simulink model "Hybrid_BCI"  (Simulink 8.6)
settings: Solver=FixedStepDiscrete  StartTime=0.0  StopTime=260  FixedStep=1/256  RelTol=1e-3
undefined symbols (not defined in the file or in its folder): currentCFG_Hybrid_BCI_UB, UB
libraries: dspstat3 x6, gRTanalyze x5, dspbuff3 x5, simulink x2, Tools x1, instrumentlib x1, gUSBamplib x1
Description:
  | g.USBamp based SSVEP based BCI
  | 
  | Copyright g.tec medical engineering GmbH
settings Model: Creator=g.tec medical engineering GmbH  ModifiedByFormat=g.tec  LastModifiedBy=g.tec
settings DebuggingCC: FcnCallInpInsideContextMsg=UseLocalSettings

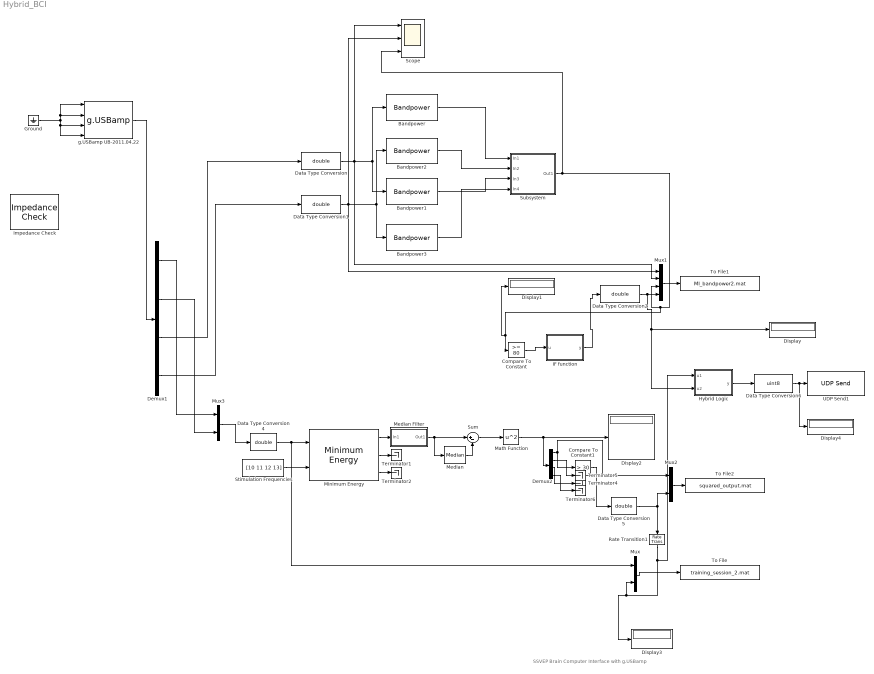
== system Hybrid_BCI ==
  note: SSVEP Brain Computer Interface with g.USBamp
  Bandpower : gRTanalyze/Bandpower  Order=5  LowerFreq=8  UpperFreq=12  WindowLength=128
  Bandpower1 : gRTanalyze/Bandpower  Order=5  LowerFreq=12  UpperFreq=30  WindowLength=128
  Bandpower2 : gRTanalyze/Bandpower  Order=5  LowerFreq=8  UpperFreq=12  WindowLength=128
  Bandpower3 : gRTanalyze/Bandpower  Order=5  LowerFreq=12  UpperFreq=30  WindowLength=128
  Compare To Constant : simulink/Logic and Bit Operations/Compare To Constant  relop=>=  const=80  OutDataTypeStr=boolean
  Compare To Constant1 : simulink/Logic and Bit Operations/Compare To Constant  relop=>  const=30  OutDataTypeStr=boolean
  Data Type Conversion{,1..2,4..5} (5 alike) : DataTypeConversion  OutDataTypeStr=double
  Data Type Conversion6 : DataTypeConversion  OutDataTypeStr=uint8
  Demux1 : Demux
  Demux2 : Demux
  Display{,1..4} (5 alike) : Display
  Ground : Ground
  Hybrid Logic : MATLAB Function  TreatAsAtomicUnit=on
  IF function : MATLAB Function  TreatAsAtomicUnit=on
  Impedance Check : Tools/Impedance Check
  Math Function : Math  Operator=square  SaturateOnIntegerOverflow=on
  Median : dspstat3/Median  sortAlg=Quick sort  directionMode=Entire input  dimension=1  outputDataTypeStr=Inherit: Same as accumulator  outputLastDataTypeStr=Inherit: Same as accumulator  outputMin=[]  outputMax=[]  accumDataTypeStr=Inherit: Same as product output  accumLastDataTypeStr=Inherit: Same as product output  roundingMode=Floor  overflowMode=off
      settings: allowOverrides=off
  Median Filter : Subsystem  mask(Moving Median Filter){buflen=10}
      mask prompts: buflen "Filter Length"
      mask help:
      | Smoothes the input channels over time by computing the median value for
      | the specified number of samples.
      mask init:
      | blockhandle = get_param(gcb,'Handle');
      | sysname = get(blockhandle,'Path');
      | syspath = [ sysname '/' ];
      | name = [ syspath get(blockhandle,'Name') ];
      | path = [ name '/' ];
      | if buflen < 3
      |   buflen = 10;
      |   set_param(name,'buflen',num2str(buflen));
      | end
      | set_param([ path 'Collect'],'siz',num2str(buflen));
      | try
      |   set_param([ path 'Collect'],'TreatMby1Signals','M channels (this choice will be removed - see release notes)');
      | catch
      | end
      mask Help:
      | Smoothes the input channels over time by computing the median value for
      | the specified number of samples.
      | 
      | Filter Length ... The length of the smoothing window in samples. (Default 10)
  Minimum Energy : gRTanalyze/Minimum Energy  bufflen=768  reprate=0.20  numharmonics=1  modelorder=7
  Mux : Mux  Inputs=2
  Mux1 : Mux
  Mux2 : Mux  Inputs=2
  Mux3 : Mux  Inputs=2
  Rate Transition1 : RateTransition
  Scope : Scope  NumInputPorts=3
  Stimulation Frequencies : Constant  Value=[10 11 12 13]  SampleTime=1/256
  Subsystem : Subsystem
  Sum : Sum  Inputs=|+-
  Terminator{1..2,4..6} (5 alike) : Terminator
  To File : ToFile  Filename=training_session_2.mat  MatrixName=y
  To File1 : ToFile  Filename=MI_bandpower2.mat  MatrixName=y
  To File2 : ToFile  Filename=squared_output.mat  MatrixName=y
  UDP Send1 : instrumentlib/UDP Send  Host=172.22.11.2  Port=1111  LocalPort=-1  EnableBlockingMode=on  ByteOrder=BigEndian
  g.USBamp UB-2011.04.22 : gUSBamplib/g.USBamp  cfg=currentCFG_Hybrid_BCI_UB-2011.04.22.cfg  snr=UB-2011.04.22
  wires:
  g.USBamp UB-2011.04.22/1 -> Demux1/1
  Ground/1 -> g.USBamp UB-2011.04.22/4, g.USBamp UB-2011.04.22/3, g.USBamp UB-2011.04.22/2, g.USBamp UB-2011.04.22/1
  Data Type Conversion/1 -> Scope/1, Mux1/1, Bandpower/1, Bandpower1/1
  Compare To Constant/1 -> IF function/1(u)
  Data Type Conversion1/1 -> Scope/2, Mux1/2, Bandpower3/1, Bandpower2/1
  Bandpower/1 -> Subsystem/1(In1)
  Bandpower2/1 -> Subsystem/2(In2)
  Bandpower1/1 -> Subsystem/3(In3)
  Bandpower3/1 -> Subsystem/4(In4)
  Mux1/1 -> To File1/1
  Subsystem/1(Out1) -> Scope/3, Display1/1, Compare To Constant/1, Mux1/3
  Data Type Conversion2/1 -> Hybrid Logic/2(u2), Display/1, Mux1/4
  IF function/1(y) -> Data Type Conversion2/1
  Stimulation Frequencies/1 -> Minimum Energy/2
  Minimum Energy/1 -> Median Filter/1(In1)
  Median Filter/1(Out1) -> Sum/1, Median/1
  Minimum Energy/2 -> Terminator1/1
  Minimum Energy/3 -> Terminator2/1
  Mux3/1 -> Data Type Conversion4/1
  Data Type Conversion4/1 -> Mux/1, Minimum Energy/1
  Mux/1 -> To File/1
  Rate Transition1/1 -> Hybrid Logic/1(u1), Mux/2, Display3/1
  Median/1 -> Sum/2
  Sum/1 -> Math Function/1
  Math Function/1 -> Demux2/1, Display2/1
  Demux2/1 -> Mux2/1, Compare To Constant1/1
  Demux2/2 -> Terminator5/1
  Demux2/3 -> Terminator4/1
  Demux2/4 -> Terminator6/1
  Compare To Constant1/1 -> Data Type Conversion5/1
  Data Type Conversion5/1 -> Rate Transition1/1, Mux2/2
  Mux2/1 -> To File2/1
  Data Type Conversion6/1 -> Display4/1, UDP Send1/1
  Hybrid Logic/1(y) -> Data Type Conversion6/1
  Demux1/2 -> Mux3/2
  Demux1/1 -> Mux3/1
  Demux1/3 -> Data Type Conversion/1
  Demux1/4 -> Data Type Conversion1/1

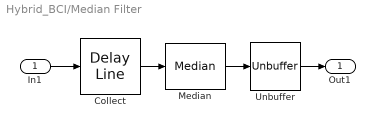
== system Hybrid_BCI/Median Filter ==
  In1 : Inport
  Collect : dspbuff3/Delay Line  siz=10  ic=0  directfeed=on  enable_output=off  hold_output=off  TreatMby1Signals=M channels (this choice will be removed - see release notes)  OutputFrames=on
  Median : dspstat3/Median  sortAlg=Quick sort  directionMode=Specified dimension  dimension=1  outputDataTypeStr=Inherit: Same as accumulator  outputLastDataTypeStr=Inherit: Same as accumulator  outputMin=[]  outputMax=[]  accumDataTypeStr=Inherit: Same as product output  accumLastDataTypeStr=Inherit: Same as product output  roundingMode=Floor  overflowMode=off
      settings: allowOverrides=off
  Unbuffer : Unbuffer
  Out1 : Outport
  wires:
  Unbuffer/1 -> Out1/1
  Median/1 -> Unbuffer/1
  Collect/1 -> Median/1
  In1/1 -> Collect/1

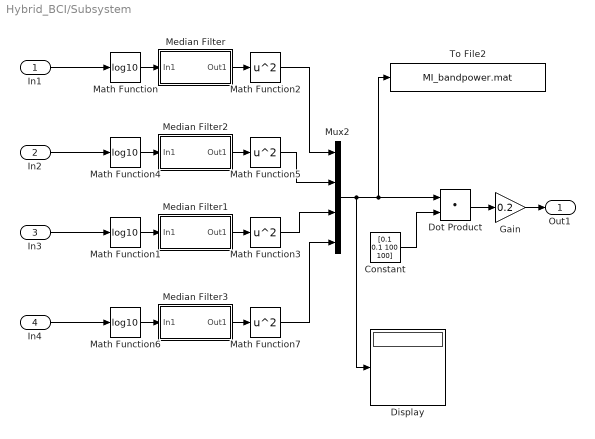
== system Hybrid_BCI/Subsystem ==
  In1 : Inport
  In2 : Inport  Port=2
  In3 : Inport  Port=3
  In4 : Inport  Port=4
  Constant : Constant  Value=[0.1 0.1 100 100]
  Display : Display
  Dot Product : DotProduct  InputSameDT=on  OutDataTypeStr=Inherit: Inherit via internal rule
  Gain : Gain  Gain=0.2
  Math Function{,1,4,6} (4 alike) : Math  Operator=log10  SaturateOnIntegerOverflow=on
  Math Function{2..3,5,7} (4 alike) : Math  Operator=square  SaturateOnIntegerOverflow=on
  Median Filter : Subsystem  mask(Moving Median Filter){buflen=50}
      mask prompts: buflen "Filter Length"
      mask help:
      | Smoothes the input channels over time by computing the median value for
      | the specified number of samples.
      mask init: same as Hybrid_BCI/Median Filter
      mask Help:
      | Smoothes the input channels over time by computing the median value for
      | the specified number of samples.
      | 
      | Filter Length ... The length of the smoothing window in samples. (Default 10)
  Median Filter1 : Subsystem  mask(Moving Median Filter){buflen=50}
      mask prompts: buflen "Filter Length"
      mask help:
      | Smoothes the input channels over time by computing the median value for
      | the specified number of samples.
      mask init: same as Hybrid_BCI/Median Filter
      mask Help:
      | Smoothes the input channels over time by computing the median value for
      | the specified number of samples.
      | 
      | Filter Length ... The length of the smoothing window in samples. (Default 10)
  Median Filter2 : Subsystem  mask(Moving Median Filter){buflen=50}
      mask prompts: buflen "Filter Length"
      mask help:
      | Smoothes the input channels over time by computing the median value for
      | the specified number of samples.
      mask init: same as Hybrid_BCI/Median Filter
      mask Help:
      | Smoothes the input channels over time by computing the median value for
      | the specified number of samples.
      | 
      | Filter Length ... The length of the smoothing window in samples. (Default 10)
  Median Filter3 : Subsystem  mask(Moving Median Filter){buflen=50}
      mask prompts: buflen "Filter Length"
      mask help:
      | Smoothes the input channels over time by computing the median value for
      | the specified number of samples.
      mask init: same as Hybrid_BCI/Median Filter
      mask Help:
      | Smoothes the input channels over time by computing the median value for
      | the specified number of samples.
      | 
      | Filter Length ... The length of the smoothing window in samples. (Default 10)
  Mux2 : Mux
  To File2 : ToFile  Filename=MI_bandpower.mat  MatrixName=y
  Out1 : Outport
  wires:
  Math Function5/1 -> Mux2/2
  Math Function3/1 -> Mux2/3
  Median Filter1/1(Out1) -> Math Function3/1
  Math Function/1 -> Median Filter/1(In1)
  Math Function2/1 -> Mux2/1
  Median Filter3/1(Out1) -> Math Function7/1
  Math Function1/1 -> Median Filter1/1(In1)
  In4/1 -> Math Function6/1
  Math Function6/1 -> Median Filter3/1(In1)
  Median Filter/1(Out1) -> Math Function2/1
  In3/1 -> Math Function1/1
  Dot Product/1 -> Gain/1
  Math Function7/1 -> Mux2/4
  Mux2/1 -> Display/1, To File2/1, Dot Product/1
  In1/1 -> Math Function/1
  In2/1 -> Math Function4/1
  Constant/1 -> Dot Product/2
  Median Filter2/1(Out1) -> Math Function5/1
  Math Function4/1 -> Median Filter2/1(In1)
  Gain/1 -> Out1/1

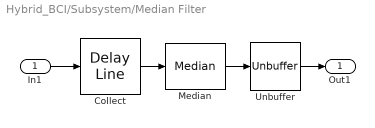
== system Hybrid_BCI/Subsystem/Median Filter ==
  In1 : Inport
  Collect : dspbuff3/Delay Line  siz=50  ic=0  directfeed=on  enable_output=off  hold_output=off  TreatMby1Signals=M channels (this choice will be removed - see release notes)  OutputFrames=on
  Median : dspstat3/Median  sortAlg=Quick sort  directionMode=Specified dimension  dimension=1  outputDataTypeStr=Inherit: Same as accumulator  outputLastDataTypeStr=Inherit: Same as accumulator  outputMin=[]  outputMax=[]  accumDataTypeStr=Inherit: Same as product output  accumLastDataTypeStr=Inherit: Same as product output  roundingMode=Floor  overflowMode=off
      settings: allowOverrides=off
  Unbuffer : Unbuffer
  Out1 : Outport
  wires:
  Unbuffer/1 -> Out1/1
  Median/1 -> Unbuffer/1
  Collect/1 -> Median/1
  In1/1 -> Collect/1

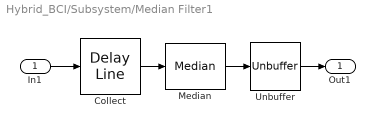
== system Hybrid_BCI/Subsystem/Median Filter1 ==
  In1 : Inport
  Collect : dspbuff3/Delay Line  siz=50  ic=0  directfeed=on  enable_output=off  hold_output=off  TreatMby1Signals=M channels (this choice will be removed - see release notes)  OutputFrames=on
  Median : dspstat3/Median  sortAlg=Quick sort  directionMode=Specified dimension  dimension=1  outputDataTypeStr=Inherit: Same as accumulator  outputLastDataTypeStr=Inherit: Same as accumulator  outputMin=[]  outputMax=[]  accumDataTypeStr=Inherit: Same as product output  accumLastDataTypeStr=Inherit: Same as product output  roundingMode=Floor  overflowMode=off
      settings: allowOverrides=off
  Unbuffer : Unbuffer
  Out1 : Outport
  wires:
  Unbuffer/1 -> Out1/1
  Median/1 -> Unbuffer/1
  Collect/1 -> Median/1
  In1/1 -> Collect/1

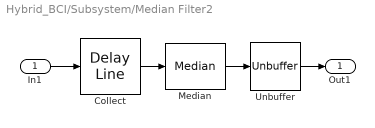
== system Hybrid_BCI/Subsystem/Median Filter2 ==
  In1 : Inport
  Collect : dspbuff3/Delay Line  siz=50  ic=0  directfeed=on  enable_output=off  hold_output=off  TreatMby1Signals=M channels (this choice will be removed - see release notes)  OutputFrames=on
  Median : dspstat3/Median  sortAlg=Quick sort  directionMode=Specified dimension  dimension=1  outputDataTypeStr=Inherit: Same as accumulator  outputLastDataTypeStr=Inherit: Same as accumulator  outputMin=[]  outputMax=[]  accumDataTypeStr=Inherit: Same as product output  accumLastDataTypeStr=Inherit: Same as product output  roundingMode=Floor  overflowMode=off
      settings: allowOverrides=off
  Unbuffer : Unbuffer
  Out1 : Outport
  wires:
  Unbuffer/1 -> Out1/1
  Median/1 -> Unbuffer/1
  Collect/1 -> Median/1
  In1/1 -> Collect/1

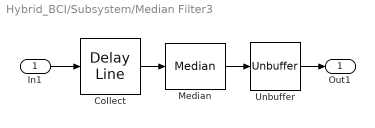
== system Hybrid_BCI/Subsystem/Median Filter3 ==
  In1 : Inport
  Collect : dspbuff3/Delay Line  siz=50  ic=0  directfeed=on  enable_output=off  hold_output=off  TreatMby1Signals=M channels (this choice will be removed - see release notes)  OutputFrames=on
  Median : dspstat3/Median  sortAlg=Quick sort  directionMode=Specified dimension  dimension=1  outputDataTypeStr=Inherit: Same as accumulator  outputLastDataTypeStr=Inherit: Same as accumulator  outputMin=[]  outputMax=[]  accumDataTypeStr=Inherit: Same as product output  accumLastDataTypeStr=Inherit: Same as product output  roundingMode=Floor  overflowMode=off
      settings: allowOverrides=off
  Unbuffer : Unbuffer
  Out1 : Outport
  wires:
  Unbuffer/1 -> Out1/1
  Median/1 -> Unbuffer/1
  Collect/1 -> Median/1
  In1/1 -> Collect/1

== matlab function Hybrid Logic ==
  data: u1 input double; y output double; u2 input double
function y = fcn(u1,u2)
%#codegen
if u1==0 && u2==0
    y=0;
elseif u1==1&&u2==2
    y=1;
elseif u1==1&&u2==0
    y=1;
else
    y=2;
end

== matlab function IF function ==
  data: u input double; y output double
function y = fcn(u)
%#codegen
if u==0
    y=0;
else
    y=2;
end
